simulink model "Simulink"  (R2023b)
settings: Solver=VariableStepAuto  StartTime=0.0  StopTime=10.0  RelTol=1e-3
libraries: fl_lib x5, nesl_utility x3, ee_lib x1
settings Model: Creator=MiguelFG  LastModifiedBy=MiguelFG

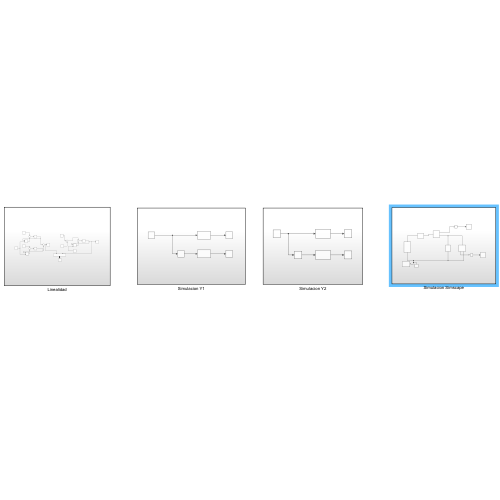
[thumbnail: Simulink's stored preview of the top-level diagram]
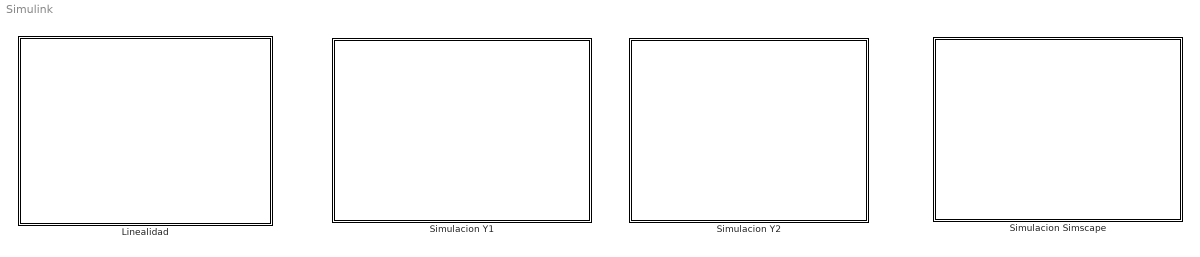
== system Simulink ==
  Linealidad : Subsystem
  Simulacion Simscape : Subsystem
  Simulacion Y1 : Subsystem
  Simulacion Y2 : Subsystem

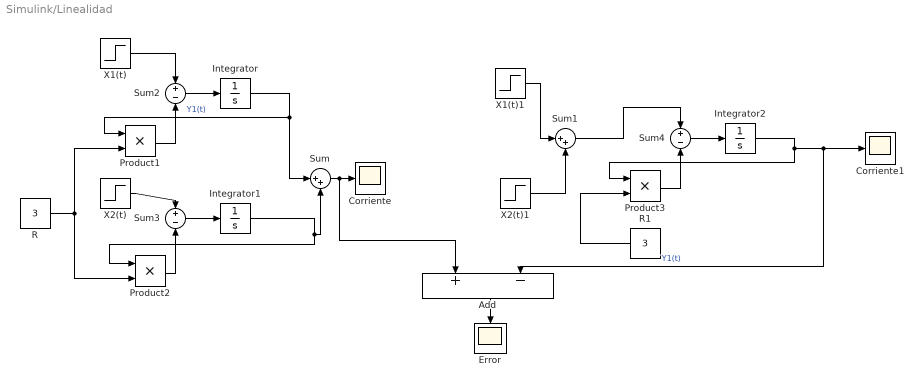
== system Simulink/Linealidad ==
  Add : Sum  Inputs=+-
  Corriente : Scope
  Corriente1 : Scope
  Error : Scope
  Integrator : Integrator
  Integrator1 : Integrator
  Integrator2 : Integrator
  Product1 : Product
  Product2 : Product
  Product3 : Product
  R : Constant  Value=3
  R1 : Constant  Value=3
  Sum : Sum  Inputs=|++
  Sum1 : Sum  Inputs=|++
  Sum2 : Sum  Inputs=+-
  Sum3 : Sum  Inputs=+-
  Sum4 : Sum  Inputs=+-
  X1(t) : Step  Time=0  After=2  SampleTime=0
  X1(t)1 : Step  Time=0  After=2  SampleTime=0
  X2(t) : Step  Time=0  SampleTime=0
  X2(t)1 : Step  Time=0  SampleTime=0
  wires:
  Product1/1 -> Sum2/2
  X1(t)1/1 -> Sum1/1
  Product2/1 -> Sum3/2
  R/1 -> Product1/2, Product2/2
  X2(t)/1 -> Sum3/1
  Sum3/1 -> Integrator1/1
  Integrator1/1 -> Product2/1, Sum/2
  Integrator2/1 -> Add/2, Corriente1/1, Product3/1  "Y1(t)"
  Integrator/1 -> Sum/1, Product1/1  "Y1(t)"
  Sum2/1 -> Integrator/1
  Product3/1 -> Sum4/2
  R1/1 -> Product3/2
  Sum4/1 -> Integrator2/1
  X2(t)1/1 -> Sum1/2
  Add/1 -> Error/1
  Sum1/1 -> Sum4/1
  X1(t)/1 -> Sum2/1
  Sum/1 -> Add/1, Corriente/1

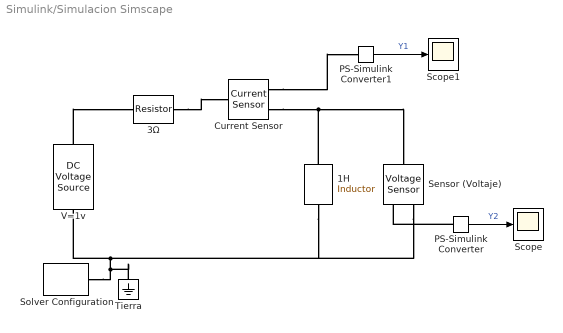
== system Simulink/Simulacion Simscape ==
  1H : ee_lib/Passive/Inductor  l=1 H  enable_L_tol=ee.enum.toleranceApplication.none  L_tol=20  tol_distribution=ee.enum.toleranceDistribution.uniform  nSigma=4  r=0 Ohm  g=1e-9 1/Ohm  enable_operating_limits=ee.enum.enable.no  operating_limit_action=ee.enum.passive.reportOpLim.warn  max_working_current=1 A  power_rating=1 W  enable_faults=ee.enum.enable.no  fault_action=simscape.enum.assert.action.none  lambdaPercent=50  k_faulted=0.9999  turnsShort=ee.enum.passive.inductor.turnsShortOption.no  openCct=ee.enum.enable.no  groundShort=ee.enum.passive.inductor.groundShortOption.no  groundShortG=0 1/Ohm  tau_fault=1e-3 s  fault_trigger=ee.enum.faults.faultTrigger.temporal  t_fault=1 s  max_permissible_voltage=100 V  n_fail_on_voltage=1  max_permissible_current=1 A  t_fail_on_current=1 s  i_L_specify=off  i_L_priority=High  i_L=0 A  i_L_nominal_specify=off  i_L_nominal_unit=A  i_L_nominal_value=1
  3Ω : fl_lib/Electrical/Electrical Elements/Resistor  R=3 Ohm  i_specify=off  i_priority=None  i=0 A  i_nominal_specify=off  i_nominal_unit=A  i_nominal_value=1  v_specify=off  v_priority=None  v=0 V  v_nominal_specify=off  v_nominal_unit=V  v_nominal_value=1
  Current Sensor : fl_lib/Electrical/Electrical Sensors/Current Sensor
  PS-Simulink Converter : nesl_utility/PS-Simulink Converter  PhysicalDomain=network_engine_domain  SubClassName=ps_output  LeftPortType=input  RightPortType=output  PseudoPeriodic=off  Frequencies=[]  VectorFormat=inherit  Unit=inherit  AffineConversion=off
  PS-Simulink Converter1 : nesl_utility/PS-Simulink Converter  PhysicalDomain=network_engine_domain  SubClassName=ps_output  LeftPortType=input  RightPortType=output  PseudoPeriodic=off  Frequencies=[]  VectorFormat=inherit  Unit=inherit  AffineConversion=off
  Scope : Scope
  Scope1 : Scope
  Sensor (Voltaje) : fl_lib/Electrical/Electrical Sensors/Voltage Sensor
  Solver Configuration : nesl_utility/Solver Configuration  PhysicalDomain=network_engine_domain  SubClassName=solver  LeftPortType=input  RightPortType=generic  Tones=[]  Harmonics=[]  SimulateNoise=off  Profile=off  UseLocalSampling=off  EnableSwitchedLinearOptims=on  FrequencyDomain=off  UseCCode=off  RelTol=0.001  AbsTol=0.001  MinStep=1e-09  ToWorkspace=off  RevertToSquareIcSolve=off  NumHomotopyIterations=100  PhasorMode=off  PhasorModeNumHarmonics=1  ConsistencySolver=NEWTON_FTOL  IndexReductionMethod=DerivativeReplacement  DoDC=off  ResidualTolerance=1e-09  ConsistencyTolSource=GLOBAL  ConsistencyAbsTol=0.001  ConsistencyRelTol=0.001  ConsistencyTolFactor=0.001  UseLocalSolver=off  LocalSolverChoice=NE_BACKWARD_EULER_ADVANCER  ResolveIndetEquations=on  FunctionEvalNumThread=1  LocalSolverSampleTime=0.001  DoFixedCost=off  MaxNonlinIter=3  MaxModeIter=2  ComputeImpulses=off  ImpulseIterations=2  LinearAlgebra=auto  LinearAlgebraNumThread=0  EquationFormulation=NE_TIME_EF  DelaysMemoryBudget=1024  AutomaticFiltering=on  FilteringTimeConstant=0.001  PartitionStorageMethod=AS_NEEDED  PartitionMemoryBudget=1024  PartitionMethod=ROBUST  MultibodyUseLocalSolver=off  MultibodyLocalSolverChoice=ODE1  MultibodyLocalSolverSampleTime=0.001
  Tierra : fl_lib/Electrical/Electrical Elements/Electrical Reference
  V=1v : fl_lib/Electrical/Electrical Sources/DC Voltage Source  v0=1 V
  wires:
  PS-Simulink Converter1/1 -> Scope1/1  "Y1"
  PS-Simulink Converter/1 -> Scope/1  "Y2"
  connections:
  V=1v/LConn1 -- 3Ω/LConn1
  Tierra/LConn1 -- Sensor (Voltaje)/RConn2 -- 1H/RConn1 -- V=1v/RConn1 -- Solver Configuration/RConn1
  Current Sensor/RConn1 -- PS-Simulink Converter1/LConn1
  1H/LConn1 -- Current Sensor/RConn2 -- Sensor (Voltaje)/LConn1
  3Ω/RConn1 -- Current Sensor/LConn1
  PS-Simulink Converter/LConn1 -- Sensor (Voltaje)/RConn1

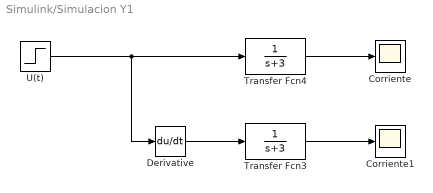
== system Simulink/Simulacion Y1 ==
  Corriente : Scope
  Corriente1 : Scope
  Derivative : Derivative
  Transfer Fcn3 : TransferFcn  Denominator=[1 3]
  Transfer Fcn4 : TransferFcn  Denominator=[1 3]
  U(t) : Step  Time=0  SampleTime=0
  wires:
  Derivative/1 -> Transfer Fcn3/1
  Transfer Fcn4/1 -> Corriente/1
  Transfer Fcn3/1 -> Corriente1/1
  U(t)/1 -> Transfer Fcn4/1, Derivative/1

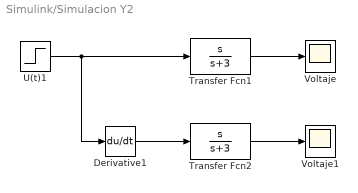
== system Simulink/Simulacion Y2 ==
  Derivative1 : Derivative
  Transfer Fcn1 : TransferFcn  Numerator=[1 0]  Denominator=[1 3]
  Transfer Fcn2 : TransferFcn  Numerator=[1 0]  Denominator=[1 3]
  U(t)1 : Step  Time=0  SampleTime=0
  Voltaje : Scope
  Voltaje1 : Scope
  wires:
  Transfer Fcn2/1 -> Voltaje1/1
  U(t)1/1 -> Transfer Fcn1/1, Derivative1/1
  Transfer Fcn1/1 -> Voltaje/1
  Derivative1/1 -> Transfer Fcn2/1
